simulink model "Medical3"  (R2019b)
settings: Solver=FixedStepAuto  StartTime=0.0  StopTime=inf  RelTol=1e-3
libraries: androiduilib x3, dspfdesign x3, androidsensorlib x1, vrlib x1
settings Model: SimulationMode=accelerator  Creator=User  LastModifiedBy=suris
settings OptimizationCC: EnhancedBackFolding=on  PassReuseOutputArgsAs=Individual arguments  ZeroExternalMemoryAtStartup=off  ZeroInternalMemoryAtStartup=off  MaxStackSize=64  OptimizeBlockOrder=speed  DifferentSizesBufferReuse=on  OptimizationCustomize=off  EfficientTunableParamExpr=on
settings DebuggingCC: ParameterTunabilityLossMsg=error
settings HardwareCC: ProdBitPerPointer=32  ProdBitPerSizeT=32  ProdBitPerPtrDiffT=32  ProdLargestAtomicInteger=Long  ProdLargestAtomicFloat=Double  ProdWordSize=32  ProdHWDeviceType=ARM Compatible->ARM Cortex  UseEmbeddedCoderFeatures=off  UseSimulinkCoderFeatures=off
settings SFSimCC: MATLABDynamicMemAlloc=off
settings RTWCC: SystemTargetFile=ert.tlc  HardwareBoard=Android Device  TLCOptions="-aInlineSetEventsForThisBaseRateFcn=TLC_FALSE -aSuppressMultiTaskScheduler=TLC_FALSE  -aRateBasedStepFcn=0"  TemplateMakefile=ert_default_tmf  GenerateReport=on  RTWVerbose=off  Toolchain=Android SDK/NDK Tools  IncludeHyperlinkInReport=on  LaunchReport=on  GenerateTraceInfo=on  GenerateTraceReport=on  GenerateTraceReportSl=on  GenerateTraceReportSf=on  GenerateTraceReportEml=on
settings CodeAppCC: ForceParamTrailComments=on  IgnoreCustomStorageClasses=off  OperatorAnnotations=on  SimulinkDataObjDesc=on  SFDataObjDesc=on  MangleLength=10  InsertBlockDesc=on
settings ERTTargetCC: SupportNonInlinedSFcns=on

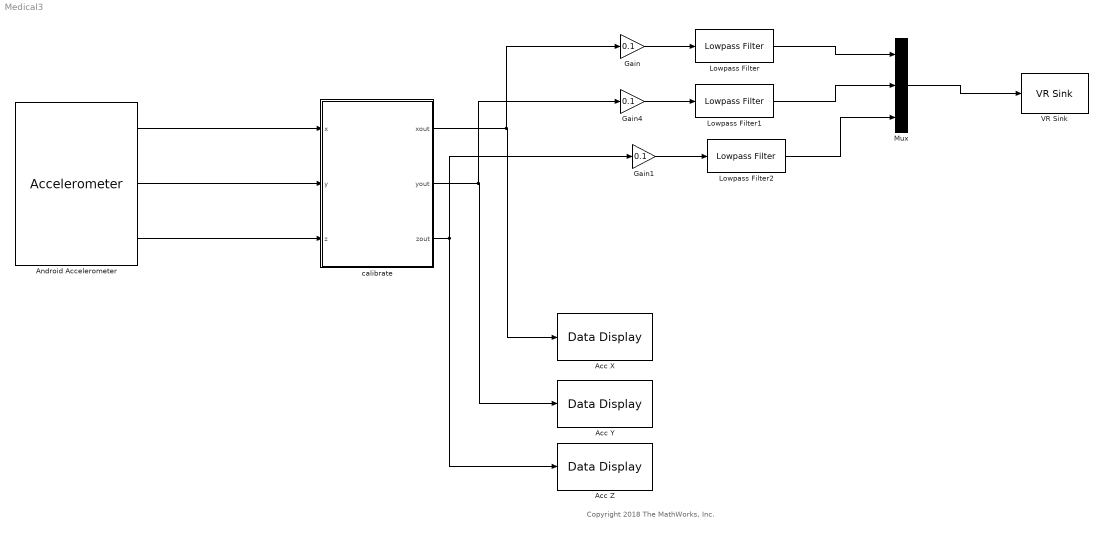
== system Medical3 ==
  note: Copyright 2018 The MathWorks, Inc.
  Acc X : androiduilib/Data Display  DataDisplayId=Medical3/Acc_X  Format=Float  Precision=6  SimulateUsing=Code generation  blockPlatform=Android
      settings: SourceProductName=Simulink Support Package for Android Devices  SourceProductBaseCode=ANDROID
  Acc Y : androiduilib/Data Display  DataDisplayId=Medical3/Acc_Y  Format=Float  Precision=6  SimulateUsing=Code generation  blockPlatform=Android
      settings: SourceProductName=Simulink Support Package for Android Devices  SourceProductBaseCode=ANDROID
  Acc Z : androiduilib/Data Display  DataDisplayId=Medical3/Acc_Z  Format=Float  Precision=6  SimulateUsing=Code generation  blockPlatform=Android
      settings: SourceProductName=Simulink Support Package for Android Devices  SourceProductBaseCode=ANDROID
  Android Accelerometer : androidsensorlib/Accelerometer  OutputVector=off  SampleTime=0.01  BlockPlatform=Android
      settings: SourceProductName=Simulink Support Package for Android Devices  SourceProductBaseCode=ANDROID
  Gain : Gain  Gain=0.1
  Gain1 : Gain  Gain=0.1
  Gain4 : Gain  Gain=0.1
  Lowpass Filter : dspfdesign/Lowpass Filter  FilterType=FIR  DesignForMinimumOrder=on  FilterOrder=50  PassbandFrequency=2  StopbandFrequency=6  PassbandRipple=0.1  StopbandAttenuation=40  InheritSampleRate=off  SampleRate=100  SimulateUsing=Interpreted execution  roundingMode=Floor  coeffsDataTypeStr=fixdt(1,16)
  Lowpass Filter1 : dspfdesign/Lowpass Filter  FilterType=FIR  DesignForMinimumOrder=on  FilterOrder=50  PassbandFrequency=2  StopbandFrequency=6  PassbandRipple=0.1  StopbandAttenuation=40  InheritSampleRate=off  SampleRate=100  SimulateUsing=Interpreted execution  roundingMode=Floor  coeffsDataTypeStr=fixdt(1,16)
  Lowpass Filter2 : dspfdesign/Lowpass Filter  FilterType=FIR  DesignForMinimumOrder=on  FilterOrder=50  PassbandFrequency=2  StopbandFrequency=6  PassbandRipple=0.1  StopbandAttenuation=40  InheritSampleRate=off  SampleRate=100  SimulateUsing=Interpreted execution  roundingMode=Floor  coeffsDataTypeStr=fixdt(1,16)
  Mux : Mux  Inputs=3
  VR Sink : vrlib/VR Sink  InstantiateOnLoad=on  SampleTime=0.1  ViewEnable=on  RemoteChange=off  RemoteView=off  FieldsWritten=cursor.translation.3.1.1.double  WorldFileName=8_palline_color.wrl  AutoView=off  VideoDimensions=[]  AllowVariableSize=off  FigureProperties="{'Position', 'Name', 'Viewpoint', 'CameraBound', 'CameraDirection', 'CameraPosition', 'CameraUpVector', 'ZoomFactor', 'Antialiasing', 'Headlight', 'Lighting', 'NavPanel', 'Sound', 'StatusBar', 'Stereo3D', 'Stereo3DCameraOffset', 'Stereo3DHIT', 'ToolBar', 'Textures', 'Transparency', 'Triad', 'Wireframe', 'NavZones', 'NavMode', 'NavSpeed', 'CaptureFileFormat', 'CaptureFileName', 'Record2DCompressMethod', 'Record2DCompressQuality', 'Record2D', 'Record2DFileName', 'Record2DFPS'; [5.0000000000000000e+00   9.2000000000000000e+01   5.7600000000000000e+02   3.5000000000000000e+02], '', '_untitled_1', 'on', [0.0000000000000000e+00   0.0000000000000000e+00  -1.0000000000000000e+00], [0.0000000000000000e+00   0.0000000000000000e+00   0.0000000000000000e+00], [0.0000000000000000e+00   1.0000000000000000e+00   0.0000000000000000e+00], [1.0000000000000000e+00], 'on', 'on', 'on', 'halfbar', 'on', 'on', 'off', [1.0000000149011612e-01], [0.0000000000000000e+00], 'on', 'on', 'on', 'none', 'off', 'off', 'fly', 'normal', 'tif', '%f_anim_%n.tif', 'auto', [7.5000000000000000e+01], 'off', '%f_anim_%n.avi', 'auto'}"
      settings: SourceProductName=Simulink
  calibrate : MATLAB Function  TreatAsAtomicUnit=on
  wires:
  Android Accelerometer/3 -> calibrate/3(z)
  calibrate/2(yout) -> Gain4/1, Acc Y/1
  Android Accelerometer/2 -> calibrate/2(y)
  calibrate/1(xout) -> Gain/1, Acc X/1
  calibrate/3(zout) -> Acc Z/1, Gain1/1
  Android Accelerometer/1 -> calibrate/1(x)
  Gain/1 -> Lowpass Filter/1
  Gain4/1 -> Lowpass Filter1/1
  Gain1/1 -> Lowpass Filter2/1
  Lowpass Filter/1 -> Mux/1
  Lowpass Filter1/1 -> Mux/2
  Lowpass Filter2/1 -> Mux/3
  Mux/1 -> VR Sink/1

== matlab function Medical3/calibrate ==
  data: x input single size=[1 1]; xout output size=[1 1]; y input single size=[1 1]; z input single size=[1 1]; yout output; zout output
function [xout,yout,zout] = calibrate(x,y,z)%#codegen
% calibrate - Static calibration of the accelerometer for an
% Android device. 

% Copyright 2017 The MathWorks, Inc.

calibrationstr = coder.load('slexHARAndroidCalibrationMatrix.mat');
calibrationMatrix = coder.const(calibrationstr.AndroidCalibrationMatrix);

out = [x,y,z,1]*calibrationMatrix;
xout = out(1);
yout = out(2);
zout = out(3);
